simulink model "LADRC_24aV2"  (R2024b)
settings: Solver=VariableStepAuto  StartTime=0  StopTime=50  FixedStep=0.001  RelTol=1e-5
model workspace (MAT data in the model file):
  Amp = 0.0011
  P = 0
values from neighbouring files (symbols this model uses):
  a = (1/Ms)*(bs+((Ke^2)/Rs))    (= 370.38637037)    [InitialParameter.m]
  A1 = 3.1416e-04    (= 0.00031416)    [InitialParameter.m]    (also in pneumatic_code.m = 0.000314159265359)
  A2 = 2.6389e-04    (= 0.00026389)    [InitialParameter.m]    (also in pneumatic_code.m = 0.000263893782902)
  Ar = 0.00005026    (= 5.026e-05)    [InitialParameter.m]    (also in pneumatic_code.m = 5.02654824574e-05)
  b = 1    [InitialParameter.m]    (also in pneumatic_code.m = 0.0025)
  beta = 50    [InitialParameter.m]
  ep = 0.0024    [InitialParameter.m]    (also in pneumatic_code.m = 0.02)
  g1 = 9    [InitialParameter.m]    (also in pneumatic_code.m = 10)
  g2 = 4    [InitialParameter.m]    (also in pneumatic_code.m = 9)
  g3 = 18    [InitialParameter.m]    (also in pneumatic_code.m = 5)
  g4 = 0.32    [InitialParameter.m]    (also in pneumatic_code.m = 3)
  g5 = 3    [pneumatic_code.m]
  k1 = wc^4    (= 81450625)    [InitialParameter.m]    (also in pneumatic_code.m = 3620506.28125)
  k2 = 4*wc^3    (= 3429500)    [InitialParameter.m]    (also in pneumatic_code.m = 883050.3125)
  k3 = 6*wc^2    (= 54150)    [InitialParameter.m]    (also in pneumatic_code.m = 86151.25)
  k4 = 4*wc    (= 380)    [InitialParameter.m]    (also in pneumatic_code.m = 4202.5)
  k5 = 5*(wc)    (= 102.5)    [pneumatic_code.m]
  Ke = 50    [InitialParameter.m]
  M = 0.1    [InitialParameter.m]    (also in pneumatic_code.m)
  Ms = 0.5    [InitialParameter.m]    (also in pneumatic_code.m)
  Pa = 101352    [InitialParameter.m]
  Rs = 13.5    [InitialParameter.m]    (also in pneumatic_code.m)
  wall_force = 1e12    (= 1000000000000)    [InitialParameter.m]
  WallPos = 0.1    [InitialParameter.m]
undefined symbols (not defined in the file or in its folder): L1, L2, L3
settings Model: Creator=ply  LastModifiedBy=pangl
settings OptimizationCC: ZeroExternalMemoryAtStartup=off  ZeroInternalMemoryAtStartup=off
settings DebuggingCC: UnderSpecifiedDimensionMsg=warning
settings RTWCC: TargetLang=C++
settings GRTTargetCC: TargetLangStandard=C++11 (ISO)  CodeInterfacePackaging=C++ class

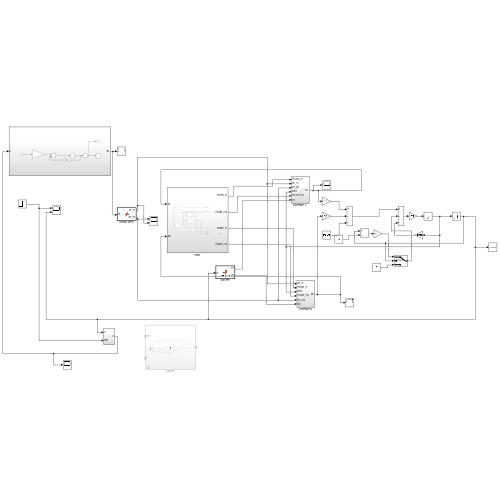
[thumbnail: Simulink's stored preview of the top-level diagram]
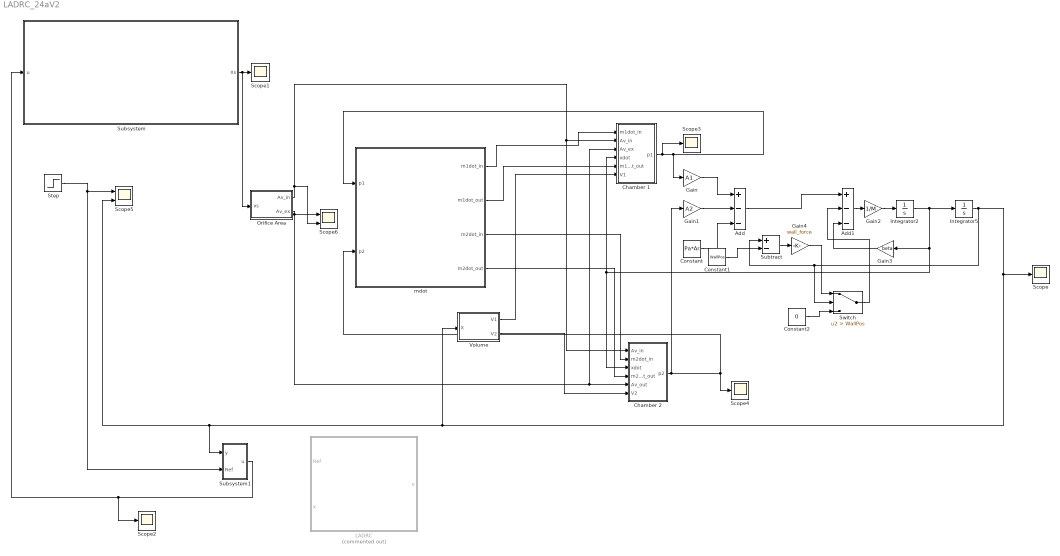
== system LADRC_24aV2 ==
  Add : Sum  Inputs=+--
  Add1 : Sum  Inputs=+--
  "Chamber 1 " : Subsystem
  Chamber 2 : Subsystem
  Constant : Constant  Value=Pa*Ar
  Constant1 : Constant  Value=WallPos
  Constant2 : Constant  Value=0
  Gain : Gain  Gain=A1
  Gain1 : Gain  Gain=A2
  Gain2 : Gain  Gain=1/M
  Gain3 : Gain  Gain=beta
  Gain4 : Gain  Gain=wall_force
  Integrator2 : Integrator
  Integrator5 : Integrator  InitialCondition=1e-4  LimitOutput=on  UpperSaturationLimit=0.15  LowerSaturationLimit=1e-4
  LADRC : Subsystem  Commented=on
  Orifice Area : MATLAB Function  TreatAsAtomicUnit=on
  Scope{,1..4} (5 alike) : Scope
  Scope5 : Scope  NumInputPorts=2
  Scope6 : Scope  NumInputPorts=2
  Step : Step  Time=0  After=0.05  SampleTime=0
  Subsystem : Subsystem
  Subsystem1 : Subsystem
  Subtract : Sum  Inputs=+-
  Switch : Switch  Criteria=u2 > Threshold  Threshold=WallPos  SaturateOnIntegerOverflow=off  InputSameDT=off
  Volume : MATLAB Function  TreatAsAtomicUnit=on
  mdot : Subsystem
  wires:
  Integrator2/1 -> Gain3/1, Chamber 2/3(xdot), "Chamber 1 "/4(xdot), Integrator5/1
  "Chamber 1 "/1(p1) -> mdot/1(p1), Gain/1, Scope3/1
  Orifice Area/1(Av_in) -> Scope6/2, Chamber 2/1(Av_in), "Chamber 1 "/2(Av_in)
  Orifice Area/2(Av_ex) -> "Chamber 1 "/3(Av_ex), Chamber 2/5(Av_out), Scope6/1
  Chamber 2/1(p2) -> Scope4/1, mdot/2(p2), Gain1/1
  Volume/1(V1) -> "Chamber 1 "/6(V1)
  Volume/2(V2) -> Chamber 2/6(V2)
  Subsystem/1(Xs) -> Orifice Area/1(xs), Scope1/1
  mdot/1(m1dot_in) -> "Chamber 1 "/1(m1dot_in)
  mdot/2(m1dot_out) -> "Chamber 1 "/5(m1dot_out)
  mdot/3(m2dot_in) -> Chamber 2/2(m2dot_in)
  mdot/4(m2dot_out) -> Chamber 2/4(m2dot_out)
  Integrator5/1 -> Switch/2, Subtract/1, Scope/1, Subsystem1/1(y), Scope5/2, Volume/1(X)
  Step/1 -> Subsystem1/2(Ref), Scope5/1
  Subsystem1/1(u) -> Scope2/1, Subsystem/1(u)
  Gain/1 -> Add/1
  Gain1/1 -> Add/2
  Constant/1 -> Add/3
  Gain2/1 -> Integrator2/1
  Add/1 -> Add1/1
  Gain3/1 -> Add1/3
  Add1/1 -> Gain2/1
  Constant1/1 -> Subtract/2
  Subtract/1 -> Gain4/1
  Gain4/1 -> Switch/1
  Constant2/1 -> Switch/3
  Switch/1 -> Add1/2

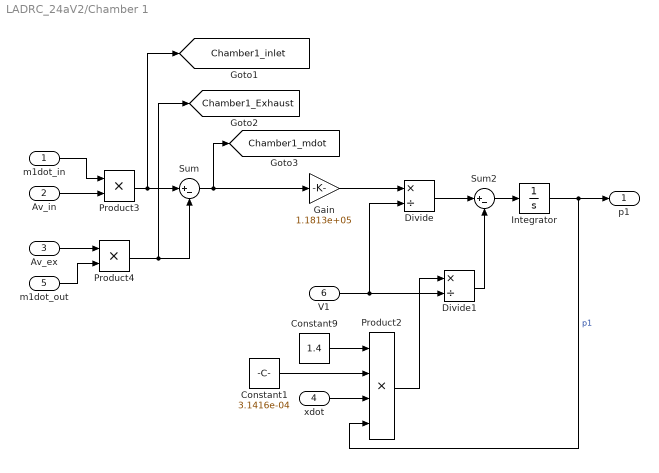
== system LADRC_24aV2/Chamber 1  ==
  m1dot_in : Inport
  Av_in : Inport  Port=2
  Av_ex : Inport  Port=3
  xdot : Inport  Port=4
  m1dot_out : Inport  Port=5
  V1 : Inport  Port=6
  Constant1 : Constant  Value=3.1416e-04
  Constant9 : Constant  Value=1.4
  Divide : Product  Inputs=*/
  Divide1 : Product  Inputs=*/
  Gain : Gain  Gain=1.1813e+05
  Integrator : Integrator  InitialCondition=101352  UpperSaturationLimit=758423  LowerSaturationLimit=101352
  Product2 : Product  Inputs=4
  Product3 : Product
  Product4 : Product
  Sum : Sum  Inputs=|+-
  Sum2 : Sum  Inputs=|+-
  p1 : Outport
  tag scope: Chamber1_Exhaust=global, Chamber1_inlet=global, Chamber1_mdot=global
  wires:
  Divide/1 -> Sum2/1
  Sum/1 -> [Chamber1_mdot], Gain/1
  Gain/1 -> Divide/1
  Divide1/1 -> Sum2/2
  Constant9/1 -> Product2/1
  Product2/1 -> Divide1/1
  Integrator/1 -> p1/1, Product2/4  "p1"
  Sum2/1 -> Integrator/1
  m1dot_in/1 -> Product3/1
  xdot/1 -> Product2/3
  Product4/1 -> [Chamber1_Exhaust], Sum/2
  Av_in/1 -> Product3/2
  Product3/1 -> [Chamber1_inlet], Sum/1
  m1dot_out/1 -> Product4/2
  Av_ex/1 -> Product4/1
  Constant1/1 -> Product2/2
  V1/1 -> Divide/2, Divide1/2

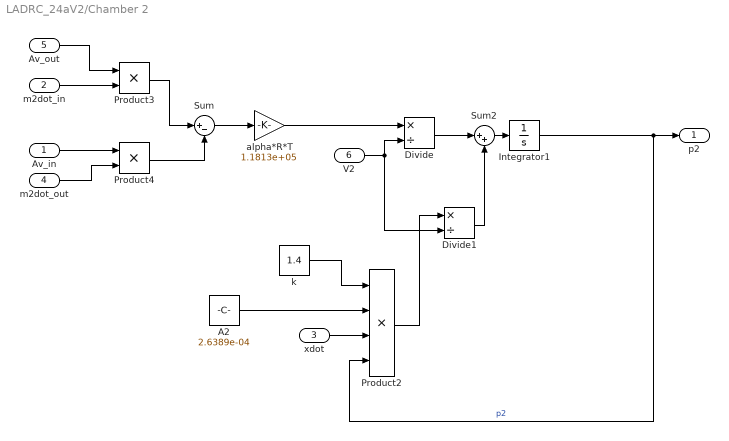
== system LADRC_24aV2/Chamber 2 ==
  Av_in : Inport
  m2dot_in : Inport  Port=2
  xdot : Inport  Port=3
  m2dot_out : Inport  Port=4
  Av_out : Inport  Port=5
  V2 : Inport  Port=6
  A2 : Constant  Value=2.6389e-04
  Divide : Product  Inputs=*/
  Divide1 : Product  Inputs=*/
  Integrator1 : Integrator  InitialCondition=10135  UpperSaturationLimit=75842  LowerSaturationLimit=10135
  Product2 : Product  Inputs=4
  Product3 : Product
  Product4 : Product
  Sum : Sum  Inputs=|+-
  Sum2 : Sum  Inputs=|++
  alpha*R*T : Gain  Gain=1.1813e+05
  k : Constant  Value=1.4
  p2 : Outport
  wires:
  m2dot_out/1 -> Product4/2
  xdot/1 -> Product2/3
  Sum2/1 -> Integrator1/1
  Integrator1/1 -> p2/1, Product2/4  "p2"
  Product2/1 -> Divide1/1
  k/1 -> Product2/1
  Divide1/1 -> Sum2/2
  A2/1 -> Product2/2
  alpha*R*T/1 -> Divide/1
  Sum/1 -> alpha*R*T/1
  Divide/1 -> Sum2/1
  Av_in/1 -> Product4/1
  m2dot_in/1 -> Product3/2
  Product3/1 -> Sum/1
  Av_out/1 -> Product3/1
  Product4/1 -> Sum/2
  V2/1 -> Divide/2, Divide1/2

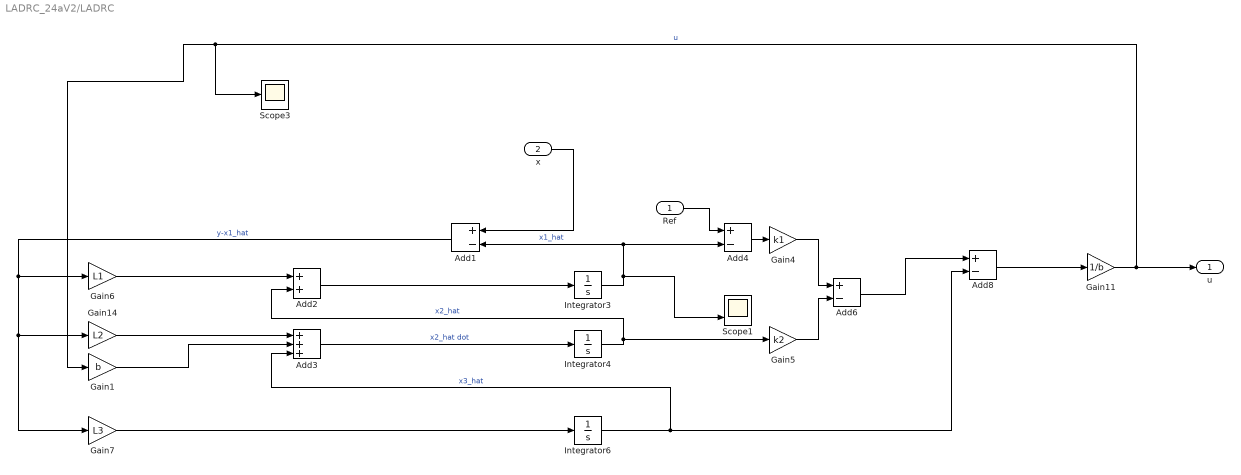
== system LADRC_24aV2/LADRC ==
  Ref : Inport
  x : Inport  Port=2
  Add{1,4,6,8} (4 alike) : Sum  Inputs=+-
  Add2 : Sum
  Add3 : Sum  Inputs=+++
  Gain1 : Gain  Gain=b
  Gain11 : Gain  Gain=1/b
  Gain14 : Gain  Gain=L2
  Gain4 : Gain  Gain=k1
  Gain5 : Gain  Gain=k2
  Gain6 : Gain  Gain=L1
  Gain7 : Gain  Gain=L3
  Integrator3 : Integrator
  Integrator4 : Integrator
  Integrator6 : Integrator
  Scope1 : Scope  NumInputPorts=2
  Scope3 : Scope
  u : Outport
  wires:
  Integrator6/1 -> Add8/2, Add3/3  "x3_hat"
  Gain5/1 -> Add6/2
  Add3/1 -> Integrator4/1  "x2_hat dot"
  Gain1/1 -> Add3/2
  Gain7/1 -> Integrator6/1
  Gain14/1 -> Add3/1
  Add2/1 -> Integrator3/1
  Integrator4/1 -> Add2/2, Gain5/1  "x2_hat"
  Add6/1 -> Add8/1
  Add8/1 -> Gain11/1
  Add4/1 -> Gain4/1
  Integrator3/1 -> Add4/2, Add1/2, Scope1/2  "x1_hat"
  Gain11/1 -> u/1, Gain1/1, Scope3/1  "u"
  Gain6/1 -> Add2/1
  Gain4/1 -> Add6/1
  Ref/1 -> Add4/1
  Add1/1 -> Gain6/1, Gain7/1, Gain14/1  "y-x1_hat"
  x/1 -> Add1/1

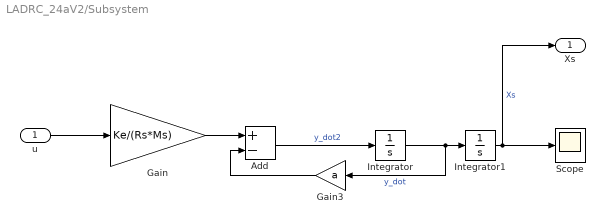
== system LADRC_24aV2/Subsystem ==
  u : Inport
  Add : Sum  Inputs=+-
  Gain : Gain  Gain=Ke/(Rs*Ms)
  Gain3 : Gain  Gain=a
  Integrator : Integrator
  Integrator1 : Integrator  LimitOutput=on  UpperSaturationLimit=0.0011  LowerSaturationLimit=-0.0011
  Scope : Scope
  Xs : Outport
  wires:
  Gain3/1 -> Add/2
  Gain/1 -> Add/1
  Add/1 -> Integrator/1  "y_dot2"
  Integrator1/1 -> Scope/1, Xs/1  "Xs"
  Integrator/1 -> Gain3/1, Integrator1/1  "y_dot"
  u/1 -> Gain/1

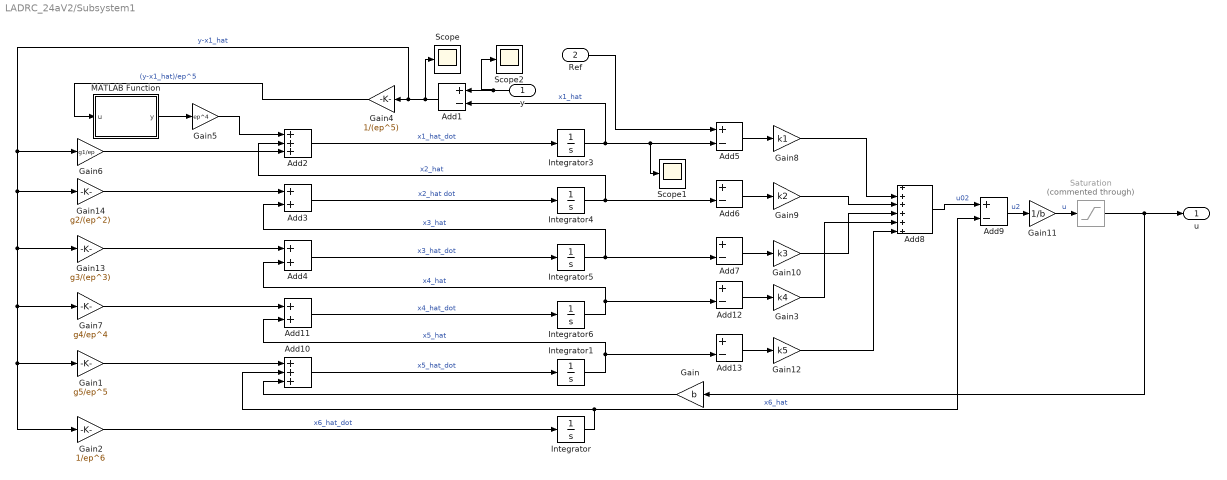
== system LADRC_24aV2/Subsystem1 ==
  y : Inport
  Ref : Inport  Port=2
  Add{1,5..7,9,12..13} (7 alike) : Sum  Inputs=+-
  Add10 : Sum  Inputs=+++
  Add11 : Sum
  Add2 : Sum  Inputs=+++
  Add3 : Sum
  Add4 : Sum
  Add8 : Sum  Inputs=++++++
  Gain : Gain  Gain=b
  Gain1 : Gain  Gain=g5/ep^5
  Gain10 : Gain  Gain=k3
  Gain11 : Gain  Gain=1/b
  Gain12 : Gain  Gain=k5
  Gain13 : Gain  Gain=g3/(ep^3)
  Gain14 : Gain  Gain=g2/(ep^2)
  Gain2 : Gain  Gain=1/ep^6
  Gain3 : Gain  Gain=k4
  Gain4 : Gain  Gain=1/(ep^5)
  Gain5 : Gain  Gain=ep^4
  Gain6 : Gain  Gain=g1/ep
  Gain7 : Gain  Gain=g4/ep^4
  Gain8 : Gain  Gain=k1
  Gain9 : Gain  Gain=k2
  Integrator{,1,4..6} (5 alike) : Integrator
  Integrator3 : Integrator  LimitOutput=on  UpperSaturationLimit=0.15  LowerSaturationLimit=1e-4
  MATLAB Function : MATLAB Function  TreatAsAtomicUnit=on
  Saturation : Saturate  Commented=through  UpperLimit=5  LowerLimit=-5
  Scope : Scope
  Scope1 : Scope
  Scope2 : Scope
  u : Outport
  wires:
  Add12/1 -> Gain3/1
  Add6/1 -> Gain9/1
  Integrator3/1 -> Add1/2, Scope1/1, Add5/2  "x1_hat"
  Integrator4/1 -> Add6/2, Add2/2  "x2_hat"
  Integrator1/1 -> Add13/2, Add11/2  "x5_hat"
  Gain12/1 -> Add8/6
  Add13/1 -> Gain12/1
  Gain1/1 -> Add10/1
  Integrator/1 -> Add9/2, Add10/2  "x6_hat"
  Gain/1 -> Add10/3
  Gain7/1 -> Add11/1
  Gain5/1 -> Add2/1
  Gain11/1 -> Saturation/1  "u"
  Gain14/1 -> Add3/1
  Add11/1 -> Integrator6/1  "x4_hat_dot"
  Ref/1 -> Add5/1
  Gain10/1 -> Add8/4
  Add4/1 -> Integrator5/1  "x3_hat_dot"
  Add1/1 -> Scope/1, Gain6/1, Gain2/1, Gain1/1, Gain7/1, Gain13/1, Gain14/1, Gain4/1  "y-x1_hat"
  Gain3/1 -> Add8/5
  Gain6/1 -> Add2/3
  Add5/1 -> Gain8/1
  Integrator5/1 -> Add7/2, Add3/2  "x3_hat"
  Add7/1 -> Gain10/1
  MATLAB Function/1(y) -> Gain5/1
  Integrator6/1 -> Add12/2, Add4/2  "x4_hat"
  Add9/1 -> Gain11/1  "u2"
  Gain8/1 -> Add8/2
  Add3/1 -> Integrator4/1  "x2_hat dot"
  Add2/1 -> Integrator3/1  "x1_hat_dot"
  y/1 -> Scope2/1, Add1/1
  Gain9/1 -> Add8/3
  Gain4/1 -> MATLAB Function/1(u)  "(y-x1_hat)/ep^5"
  Gain13/1 -> Add4/1
  Add10/1 -> Integrator1/1  "x5_hat_dot"
  Gain2/1 -> Integrator/1  "x6_hat_dot"
  Add8/1 -> Add9/1  "u02"
  Saturation/1 -> Gain/1, u/1

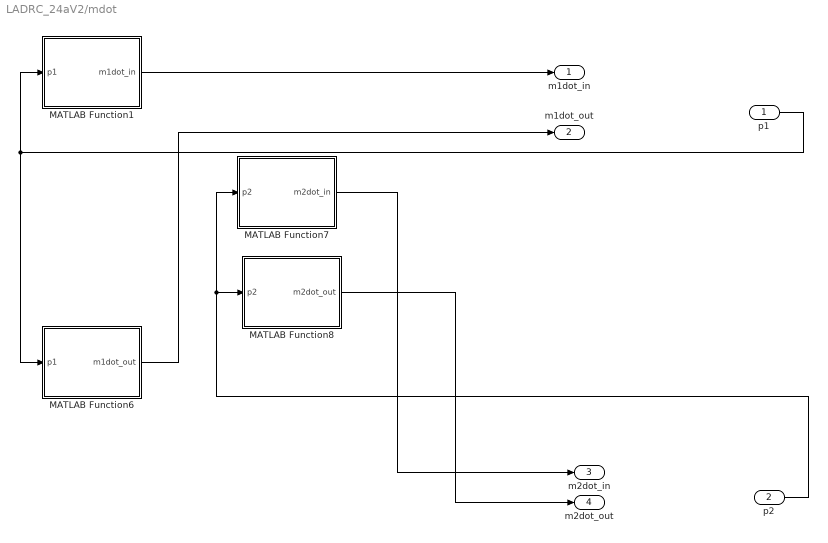
== system LADRC_24aV2/mdot ==
  p1 : Inport
  p2 : Inport  Port=2
  MATLAB Function1 : MATLAB Function  TreatAsAtomicUnit=on
  MATLAB Function6 : MATLAB Function  TreatAsAtomicUnit=on
  MATLAB Function7 : MATLAB Function  TreatAsAtomicUnit=on
  MATLAB Function8 : MATLAB Function  TreatAsAtomicUnit=on
  m1dot_in : Outport
  m1dot_out : Outport  Port=2
  m2dot_in : Outport  Port=3
  m2dot_out : Outport  Port=4
  wires:
  MATLAB Function7/1(m2dot_in) -> m2dot_in/1
  MATLAB Function6/1(m1dot_out) -> m1dot_out/1
  MATLAB Function1/1(m1dot_in) -> m1dot_in/1
  p1/1 -> MATLAB Function1/1(p1), MATLAB Function6/1(p1)
  MATLAB Function8/1(m2dot_out) -> m2dot_out/1
  p2/1 -> MATLAB Function7/1(p2), MATLAB Function8/1(p2)

== matlab function LADRC_24aV2/mdot/MATLAB Function1 ==
  data: p1 input; m1dot_in output
% function [m_dot_in,m_dot_out] = massflowrate(Avin,Avout,Pd,Pu)
% % C1 = sqrt(k/R*(2/(k+1)^((k+1)/(k-1))));
% % C2 = sqrt(2*k/(R*(k-1)));
% %Pu = 758420;
% 
% C1 = 0.0404;
% C2 = 0.1561;
% Pcr = 0.528;
% Cf=0.25;
% k = 1.4;
% T = 294;
% if (Pd/Pu)<Pcr
%     m_dot_in = Cf*Avin*C1*Pu/sqrt(T);
%     m_dot_out = Cf*Avout*C1*Pu/sqrt(T);
% elseif (Pd/Pu)>Pcr
%     m_dot_in = Cf*Avin*C2*Pu/sqrt(T)*(Pd/Pu)^(1/k)*sqrt(1-((Pd/Pu)^((k-1)/k)));
%     m_dot_out = Cf*Avout*C2*Pu/sqrt(T)*(Pd/Pu)^(1/k)*sqrt(1-((Pd/Pu)^((k-1)/k)));
% else
%     m_dot_in = 0;
%     m_dot_out = 0;
% end
% 
% 
% end

function m1dot_in = fcn(p1)
C1 = 0.0404;
C2 = 0.1561;
Pcr = 0.528;
Cf=0.25;
k = 1.4;
T = 294;
Ps=758423;      %Source Pressure
Patm=101352;    %Atmosphereic pressure
if (p1<Patm)
    p1=Patm;
elseif (p1>Ps)
    p1=Ps;
end
pu=Ps;
pd=p1;
Pratio=pd/pu;
if(Pratio <= Pcr && Pratio > 0)
    m1dot_in = Cf*C1*pu/sqrt(T);
elseif (Pratio > Pcr)
    m1dot_in = Cf*C2*pu/sqrt(T)*(pd/pu)^(1/k)*sqrt(1-(pd/pu)^((k-1)/k));
else
    m1dot_in = 0;
end

== matlab function LADRC_24aV2/Orifice Area ==
  data: xs input; Av_in output; Av_ex output
function [Av_in,Av_ex] = fcn(xs)
Xs = abs(xs);
nh = 4;
Pw = 0.0024;
Rh = 0.0019;
if (xs <= (Pw-Rh))
    Av_in=0;
elseif (xs >= (Pw+Rh))
    Av_in=pi*nh*Rh^2;
else
    temp=sqrt((Rh-Pw+xs)/(Rh+Pw-xs));
    Av_in=nh*((2*Rh*Rh*atan(temp))-((Pw-xs)*(sqrt((Rh^2)-(Pw-xs)^2))));
end

if (xs <= (-Pw-Rh))
    Av_ex=pi*nh*Rh^2;
elseif (xs >= (Rh-Pw))
    Av_ex=0;
else
    temp1=sqrt((Rh-Pw+Xs)/(Rh+Pw-Xs));
    Av_ex=nh*((2*Rh*Rh*atan(temp1))-((Pw-Xs)*(sqrt((Rh^2)-(Pw-Xs)^2))));
end
end
%

== matlab function LADRC_24aV2/Subsystem1/MATLAB Function ==
  data: u input; y output
function y = fcn(u)
%y = 0;
if u < -pi/2
    y = -(1/(4*pi));
elseif u > pi/2
    y = 1/(4*pi);
else
 y = sin(u)/(4*pi);
end

== matlab function LADRC_24aV2/Volume ==
  data: V1 output; V2 output; X input
function [V1,V2] = Volume(X)
V01 = 10e-4;
V02 = 10e-4;
L = 0.15;
A1=1.5394e-04;
A2=1.2931e-04;
% A1 = 113.1e-6;
% A2 = 95e-6;
V1 = V01+(A1*X);
V2 = V02+(A2*(L-X));

end

== matlab function LADRC_24aV2/mdot/MATLAB Function6 ==
  data: p1 input; m1dot_out output
function m1dot_out = fcn(p1)
C1 = 0.0404;
C2 = 0.1561;
Pcr = 0.528;
Cf=0.25;
k = 1.4;
T = 294;
Ps=758423;      %Source Pressure
Patm=101352;    %Atmosphereic pressure
if (p1<Patm)
    p1=Patm;
elseif (p1>Ps)
    p1=Ps;
end
pu=p1;
pd=Patm;
Pratio=pd/pu;
if(Pratio <= Pcr && Pratio > 0)
    m1dot_out = Cf*C1*pu/sqrt(T);
elseif (Pratio > Pcr)
    m1dot_out = Cf*C2*pu/sqrt(T)*(pd/pu)^(1/k)*sqrt(1-(pd/pu)^((k-1)/k));
else
    m1dot_out = 0;
end

== matlab function LADRC_24aV2/mdot/MATLAB Function7 ==
  data: p2 input; m2dot_in output
function m2dot_in = fcn(p2)
C1 = 0.0404;
C2 = 0.1561;
Pcr = 0.528;
Cf=0.25;
k = 1.4;
T = 294;
Ps=758423;      %Source Pressure
Patm=101352;    %Atmosphereic pressure
if (p2<Patm)
    p2=Patm;
elseif (p2>Ps)
    p2=Ps;
end
pu=Ps;
pd=p2;
Pratio=pd/pu;
if(Pratio <= Pcr && Pratio > 0)
    m2dot_in = Cf*C1*pu/sqrt(T);
elseif (Pratio > Pcr)
    m2dot_in = Cf*C2*pu/sqrt(T)*(pd/pu)^(1/k)*sqrt(1-(pd/pu)^((k-1)/k));
else
    m2dot_in = 0;
end

== matlab function LADRC_24aV2/mdot/MATLAB Function8 ==
  data: p2 input; m2dot_out output
function m2dot_out = fcn(p2)
C1 = 0.0404;
C2 = 0.1561;
Pcr = 0.528;
Cf=0.25;
k = 1.4;
T = 294;
Ps=758423;      %Source Pressure
Patm=101352;    %Atmosphereic pressure
if (p2<Patm)
    p2=Patm;
elseif (p2>Ps)
    p2=Ps;
end
pu=p2;
pd=Patm;
Pratio=pd/pu;
if(Pratio <= Pcr && Pratio > 0)
    m2dot_out = Cf*C1*pu/sqrt(T);
elseif (Pratio > Pcr)
    m2dot_out = Cf*C2*pu/sqrt(T)*(pd/pu)^(1/k)*sqrt(1-(pd/pu)^((k-1)/k));
else
    m2dot_out = 0;
end
